simulink model "robot"  (Simulink 7.1)
settings: Solver=ode45  StartTime=0.0  StopTime=10.0  RelTol=1e-3
undefined symbols (not defined in the file): Ts
libraries: mwblocks x8
settings Model: Creator=Bob  LastModifiedBy=Bob
settings OptimizationCC: BooleanDataType=off
settings DebuggingCC: SaveWithParameterizedLinksMsg=none  SignalResolutionControl=TryResolveAllWithWarning  SolverPrmCheckMsg=none  MultiTaskDSMMsg=warning  MultiTaskCondExecSysMsg=none  StrictBusMsg=None
settings HardwareCC: TargetUnknown=on
settings RTWCC: IncludeERTFirstTime=on
settings GRTTargetCC: TargetFcnLib=ansi_tfl_tmw.mat  ModelReferenceCompliant=off  MatFileLogging=off

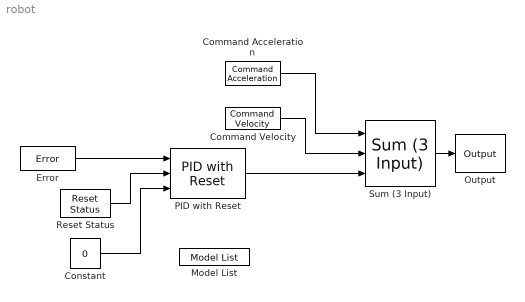
== system robot ==
  Command Acceleration : mwblocks/Command Acceleration  Tag=TCACCEL  SystemSampleTime=-1  meiAxis=.  SubSample=0  User0=0  User1=0
  Command Velocity : mwblocks/Command Velocity  Tag=TCVEL  SystemSampleTime=-1  meiAxis=.  SubSample=0  User0=0  User1=0
  Constant : Constant  Tag=CONSTANT  Value=0  OutDataType=sfix(16)  OutScaling=2^0
  Error : mwblocks/Error  Tag=ERROR  SystemSampleTime=-1  meiAxis=.  SubSample=0  User0=0  User1=0
  Model List : mwblocks/Model List  Tag=MODEL_LIST  Description=List of model numbers to load this model  SystemSampleTime=-1  meiModelList=6-11
  "Output " : mwblocks/Output   Tag=OUTPUT  SystemSampleTime=-1  meiMotor=.  SubSample=0  User0=0  User1=0
  PID with Reset : mwblocks/PID with Reset  Tag=PID_R  Description=PID with integration limit and derivative smoothing.  SystemSampleTime=-1  Kp=0.1  Ki=0  Kd=1.0  Ksm=0  Imax=0  Ts=Ts  SubSample=0  User0=0  User1=0
  Reset Status : mwblocks/Reset Status  Tag=STATUS  SystemSampleTime=-1  meiAxis=0  Enable=0  SubSample=0  User0=0  User1=0
  Sum (3 Input) : mwblocks/Sum (3 Input)  Tag=SUM  Description=3 Input sum with gains on each input  SystemSampleTime=-1  K1=125  K2=.15  K3=1  SubSample=0  User0=0  User1=0
  wires:
  Constant/1 -> PID with Reset/3
  Reset Status/1 -> PID with Reset/2
  Error/1 -> PID with Reset/1
  Sum (3 Input)/1 -> "Output "/1
  PID with Reset/1 -> Sum (3 Input)/3
  Command Acceleration/1 -> Sum (3 Input)/1
  Command Velocity/1 -> Sum (3 Input)/2
